simulink model "Control_sis_no_lineal_punto_operacion_con_observador"  (R2016a)
settings: Solver=VariableStepAuto  StartTime=0.0  StopTime=10.0  RelTol=1e-3
values from neighbouring files (symbols this model uses):
  ki = kt(:,3:3)    [ejemplodiscretro.m]
  kp = kt(:,1:2)    [ejemplodiscretro.m]
undefined symbols (not defined in the file or in its folder): A, B, C, h
settings Model: Creator=Daniel  LastModifiedBy=Daniel

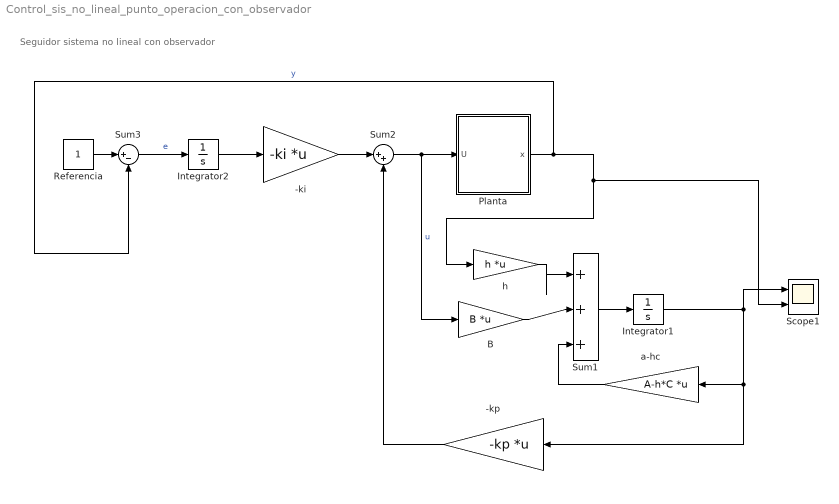
== system Control_sis_no_lineal_punto_operacion_con_observador ==
  note: Seguidor sistema no lineal con observador
  -ki : Gain  Gain=-ki  Multiplication=Matrix(K*u) (u vector)
  -kp : Gain  Gain=-kp  Multiplication=Matrix(K*u) (u vector)
  B : Gain  Gain=B  Multiplication=Matrix(K*u) (u vector)
  Integrator1 : Integrator
  Integrator2 : Integrator
  Planta : Subsystem
  Referencia : Constant
  Scope1 : Scope  NumInputPorts=2
  Sum1 : Sum  Inputs=|+++
  Sum2 : Sum  Inputs=|++
  Sum3 : Sum  Inputs=|+-
  a-hc : Gain  Gain=A-h*C  Multiplication=Matrix(K*u) (u vector)
  h : Gain  Gain=h  Multiplication=Matrix(K*u) (u vector)
  wires:
  Sum1/1 -> Integrator1/1
  a-hc/1 -> Sum1/3
  B/1 -> Sum1/2
  h/1 -> Sum1/1
  Planta/1(x) -> Sum3/2, Scope1/2, h/1  "y"
  Sum2/1 -> Planta/1(U), B/1  "u"
  Integrator2/1 -> -ki/1
  Sum3/1 -> Integrator2/1  "e"
  Referencia/1 -> Sum3/1
  -ki/1 -> Sum2/1
  Integrator1/1 -> Scope1/1, -kp/1, a-hc/1
  -kp/1 -> Sum2/2

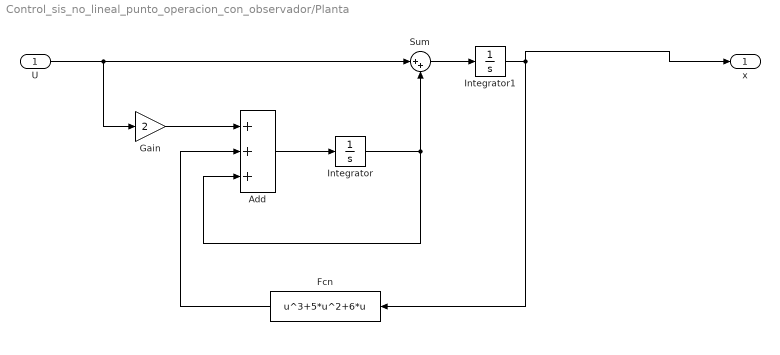
== system Control_sis_no_lineal_punto_operacion_con_observador/Planta ==
  U : Inport
  Add : Sum  Inputs=+++
  Fcn : Fcn  Expr=u^3+5*u^2+6*u
  Gain : Gain  Gain=2
  Integrator : Integrator
  Integrator1 : Integrator
  Sum : Sum  Inputs=|++
  x : Outport
  wires:
  Sum/1 -> Integrator1/1
  Add/1 -> Integrator/1
  Gain/1 -> Add/1
  Fcn/1 -> Add/2
  U/1 -> Gain/1, Sum/1
  Integrator1/1 -> Fcn/1, x/1
  Integrator/1 -> Sum/2, Add/3
